simulink model "CHB_3phaseCL_SVPWM_Phaseshift"  (R2015a)
settings: Solver=ode45  StartTime=0.0  StopTime=0.2  MaxStep=0.00001  MinStep=0.000001  RelTol=1e-3
libraries: powerlib x33, powerlib_meascontrol x3, simulink x3
settings Model: Creator=hp  LastModifiedBy=hp
settings SolverCC: ZeroCrossControl=DisableAll

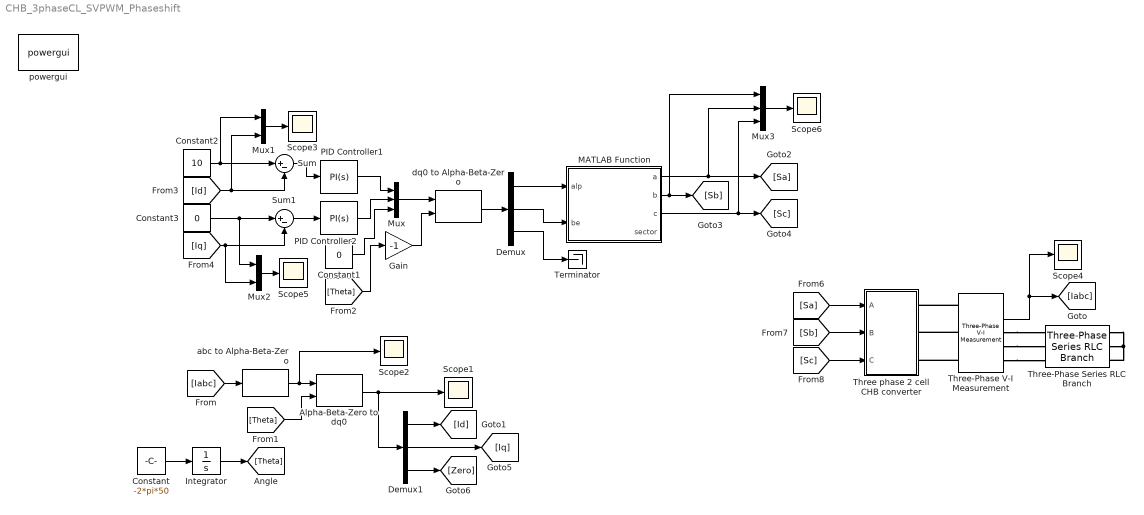
== system CHB_3phaseCL_SVPWM_Phaseshift ==
  Alpha-Beta-Zero to dq0 : powerlib_meascontrol/Transformations/Alpha-Beta-Zero to dq0  Alignment=Aligned with phase A axis
  Constant : Constant  Value=-2*pi*50
  Constant1 : Constant  Value=0
  Constant2 : Constant  Value=10
  Constant3 : Constant  Value=0
  Demux : Demux  Outputs=3
  Demux1 : Demux  Outputs=3
  Gain : Gain  Gain=-1
  Integrator : Integrator
  MATLAB Function : MATLAB Function  TreatAsAtomicUnit=on
  Mux : Mux  Inputs=3
  Mux1 : Mux  Inputs=2
  Mux2 : Mux  Inputs=2
  Mux3 : Mux  Inputs=3
  PID Controller1 : simulink/Continuous/PID Controller  Controller=PI  TimeDomain=Continuous-time  SampleTime=-1  IntegratorMethod=Forward Euler  FilterMethod=Forward Euler  Form=Parallel  UseFilter=on  ControllerParametersSource=internal  P=1  I=3128.4128432425  D=0  N=100  InitialConditionSource=internal  InitialConditionForIntegrator=0  InitialConditionForFilter=0  ExternalReset=none  LimitOutput=off  UpperSaturationLimit=inf  LowerSaturationLimit=-inf  LinearizeAsGain=on  AntiWindupMode=none  Kb=1  TrackingMode=off  Kt=1  PParamMin=[]  PParamMax=[]  IParamMin=[]  IParamMax=[]  DParamMin=[]  DParamMax=[]  NParamMin=[]  NParamMax=[]  KbParamMin=[]  KbParamMax=[]  KtParamMin=[]  KtParamMax=[]  POutMin=[]  POutMax=[]  IOutMin=[]  IOutMax=[]  DOutMin=[]  DOutMax=[]  NOutMin=[]  NOutMax=[]  KbOutMin=[]  KbOutMax=[]  KtOutMin=[]  KtOutMax=[]  IntegratorOutMin=[]  IntegratorOutMax=[]  FilterOutMin=[]  FilterOutMax=[]  SumOutMin=[]  SumOutMax=[]  SumI1OutMin=[]  SumI1OutMax=[]  SumI2OutMin=[]  SumI2OutMax=[]  SumI3OutMin=[]  SumI3OutMax=[]  SumDOutMin=[]  SumDOutMax=[]  SaturationOutMin=[]  SaturationOutMax=[]  IntegratorContinuousStateAttributes=''  IntegratorStateMustResolveToSignalObject=off  IntegratorRTWStateStorageClass=Auto  FilterContinuousStateAttributes=''  FilterStateMustResolveToSignalObject=off  FilterRTWStateStorageClass=Auto  DifferentiatorICPrevScaledInput=0  DifferentiatorOutMin=[]  DifferentiatorOutMax=[]
  PID Controller2 : simulink/Continuous/PID Controller  Controller=PI  TimeDomain=Continuous-time  SampleTime=-1  IntegratorMethod=Forward Euler  FilterMethod=Forward Euler  Form=Parallel  UseFilter=on  ControllerParametersSource=internal  P=1  I=3128.4128432425  D=0  N=100  InitialConditionSource=internal  InitialConditionForIntegrator=0  InitialConditionForFilter=0  ExternalReset=none  LimitOutput=off  UpperSaturationLimit=inf  LowerSaturationLimit=-inf  LinearizeAsGain=on  AntiWindupMode=none  Kb=1  TrackingMode=off  Kt=1  PParamMin=[]  PParamMax=[]  IParamMin=[]  IParamMax=[]  DParamMin=[]  DParamMax=[]  NParamMin=[]  NParamMax=[]  KbParamMin=[]  KbParamMax=[]  KtParamMin=[]  KtParamMax=[]  POutMin=[]  POutMax=[]  IOutMin=[]  IOutMax=[]  DOutMin=[]  DOutMax=[]  NOutMin=[]  NOutMax=[]  KbOutMin=[]  KbOutMax=[]  KtOutMin=[]  KtOutMax=[]  IntegratorOutMin=[]  IntegratorOutMax=[]  FilterOutMin=[]  FilterOutMax=[]  SumOutMin=[]  SumOutMax=[]  SumI1OutMin=[]  SumI1OutMax=[]  SumI2OutMin=[]  SumI2OutMax=[]  SumI3OutMin=[]  SumI3OutMax=[]  SumDOutMin=[]  SumDOutMax=[]  SaturationOutMin=[]  SaturationOutMax=[]  IntegratorContinuousStateAttributes=''  IntegratorStateMustResolveToSignalObject=off  IntegratorRTWStateStorageClass=Auto  FilterContinuousStateAttributes=''  FilterStateMustResolveToSignalObject=off  FilterRTWStateStorageClass=Auto  DifferentiatorICPrevScaledInput=0  DifferentiatorOutMin=[]  DifferentiatorOutMax=[]
  Scope{1..6} (6 alike) : Scope
      Scope1 settings: YMin=-22.5  YMax=7.5
      Scope2 settings: YMin=-25  YMax=25  SaveName=ScopeData2
      Scope3 settings: YMin=-20  YMax=27.5  SaveName=ScopeData3
      Scope4 settings: YMin=-27.5  YMax=27.5  SaveName=ScopeData5
      Scope5 settings: YMin=-25  YMax=0  SaveName=ScopeData4
      Scope6 settings: YMin=-1750  YMax=1750  SaveName=ScopeData6
  Sum : Sum  Inputs=|+-
  Sum1 : Sum  Inputs=|+-
  Terminator : Terminator
  Three phase 2 cell CHB converter : Subsystem  RequirementInfo="{}  %GIDa_28e9eb3f_ab9c_4722_bfe7_30b5ff19310e"
  Three-Phase Series RLC Branch : powerlib/Elements/Three-Phase Series RLC Branch  LConnTagsString=A|B|C  RConnTagsString=A|B|C  BranchType=RLC  Resistance=10  Inductance=10e-3  Capacitance=0  Measurements=None
  Three-Phase V-I Measurement : powerlib/Measurements/Three-Phase V-I Measurement  VoltageMeasurement=phase-to-phase  SetLabelV=off  LabelV=Vabc  Vpu=off  VpuLL=off  CurrentMeasurement=yes  SetLabelI=off  LabelI=Iabc  Ipu=off  Pbase=100e6  Vbase=500e3  OutputType=Complex  PhasorSimulation=off  PSBequivalent=0
  abc to Alpha-Beta-Zero : powerlib_meascontrol/Transformations/abc to Alpha-Beta-Zero
  dq0 to Alpha-Beta-Zero : powerlib_meascontrol/Transformations/dq0 to Alpha-Beta-Zero  Alignment=Aligned with phase A axis
  powergui : powerlib/powergui  Priority=1  SimulationMode=Continuous  SolverType=Tustin/Backward Euler (TBE)  SampleTime=2e-6  frequency=60  SPID=off  DisableSnubberDevices=off  DisableRonSwitches=off  DisableVfSwitches=off  SwTol=0  DisplayEquations=off  Interpol=off  methode=off  Ts=100  FunctionMessages=off  echomessages=off  HookPort=off  EnableUseOfTLC=off  x0status=blocks  frequencyindice=0  Pbase=100e6  ErrMax=1e-4  Iterations=50  UnitsV=kV  UnitsW=MW  buscounter=0  RestoreLinks=warning  ResistiveCurrentMeasurement=off  Frange=[0:2:500]  Ylog=off  Xlog=on  ShowGrid=off  save=off  variable=ZData  structure=0  ZoomFFT=off  StartTime=0.0  cycles=1  DisplayStyle=1  fundamental=60  FreqAxis=off  MaxFrequency=1000  frequencyindicesteady=1  RmsSteady=1  display=off
  wires:
  MATLAB Function/1(a) -> Mux3/2, [Sa]
  MATLAB Function/2(b) -> Mux3/1, [Sb]
  MATLAB Function/3(c) -> Mux3/3, [Sc]
  Three-Phase V-I Measurement/2 -> Scope4/1, [Iabc]
  [Sa] -> Three phase 2 cell CHB converter/1(A)
  [Sb] -> Three phase 2 cell CHB converter/2(B)
  [Sc] -> Three phase 2 cell CHB converter/3(C)
  [Iabc] -> abc to Alpha-Beta-Zero/1
  Alpha-Beta-Zero to dq0/1 -> Demux1/1, Scope1/1
  Constant/1 -> Integrator/1
  abc to Alpha-Beta-Zero/1 -> Scope2/1, Alpha-Beta-Zero to dq0/1
  Integrator/1 -> [Theta]
  [Theta] -> Alpha-Beta-Zero to dq0/2
  Demux1/1 -> [Id]
  Demux1/2 -> [Iq]
  Demux1/3 -> [Zero]
  Demux/2 -> MATLAB Function/2(be)
  Demux/1 -> MATLAB Function/1(alp)
  dq0 to Alpha-Beta-Zero/1 -> Demux/1
  Mux/1 -> dq0 to Alpha-Beta-Zero/1
  PID Controller1/1 -> Mux/1
  PID Controller2/1 -> Mux/2
  Constant1/1 -> Mux/3
  Sum1/1 -> PID Controller2/1
  Sum/1 -> PID Controller1/1
  Constant3/1 -> Sum1/1, Mux2/1
  [Iq] -> Sum1/2, Mux2/2
  [Id] -> Mux1/2, Sum/2
  Constant2/1 -> Mux1/1, Sum/1
  Mux1/1 -> Scope3/1
  Demux/3 -> Terminator/1
  Mux2/1 -> Scope5/1
  Gain/1 -> dq0 to Alpha-Beta-Zero/2
  [Theta] -> Gain/1
  Mux3/1 -> Scope6/1
  connections:
  Three-Phase Series RLC Branch/RConn1 -- Three-Phase Series RLC Branch/RConn2 -- Three-Phase Series RLC Branch/RConn3
  Three-Phase V-I Measurement/RConn1 -- Three-Phase Series RLC Branch/LConn1
  Three-Phase V-I Measurement/RConn2 -- Three-Phase Series RLC Branch/LConn2
  Three-Phase V-I Measurement/RConn3 -- Three-Phase Series RLC Branch/LConn3
  Three-Phase V-I Measurement/LConn1 -- Three phase 2 cell CHB converter/RConn1
  Three-Phase V-I Measurement/LConn2 -- Three phase 2 cell CHB converter/RConn2
  Three-Phase V-I Measurement/LConn3 -- Three phase 2 cell CHB converter/RConn3

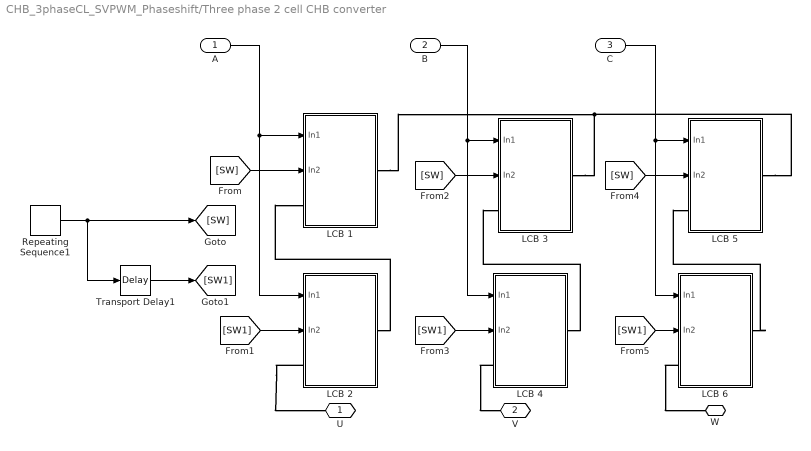
== system CHB_3phaseCL_SVPWM_Phaseshift/Three phase 2 cell CHB converter ==
  A : Inport
  B : Inport  Port=2
  C : Inport  Port=3
  LCB 1 : Subsystem
  LCB 2 : Subsystem
  LCB 3 : Subsystem
  LCB 4 : Subsystem
  LCB 5 : Subsystem
  LCB 6 : Subsystem
  Repeating Sequence1 : simulink/Sources/Repeating Sequence  rep_seq_t=[0 0.5 1]/1000  rep_seq_y=[0 1 0]
  Transport Delay1 : TransportDelay  DelayTime=1/4000
  U : PMIOPort  Port=1  Side=Right
  V : PMIOPort  Port=2  Side=Right
  W : PMIOPort  Port=3  Side=Right
  wires:
  [SW1] -> LCB 2/2(In2)
  [SW1] -> LCB 6/2(In2)
  A/1 -> LCB 2/1(In1), LCB 1/1(In1)
  [SW] -> LCB 3/2(In2)
  Repeating Sequence1/1 -> Transport Delay1/1, [SW]
  C/1 -> LCB 6/1(In1), LCB 5/1(In1)
  [SW] -> LCB 1/2(In2)
  [SW1] -> LCB 4/2(In2)
  Transport Delay1/1 -> [SW1]
  B/1 -> LCB 4/1(In1), LCB 3/1(In1)
  [SW] -> LCB 5/2(In2)
  connections:
  LCB 1/RConn1 -- LCB 5/RConn1 -- LCB 3/RConn1
  LCB 2/RConn1 -- LCB 1/LConn1
  LCB 4/RConn1 -- LCB 3/LConn1
  LCB 2/LConn1 -- U/RConn1
  LCB 6/RConn1 -- LCB 5/LConn1
  LCB 4/LConn1 -- V/RConn1
  LCB 6/LConn1 -- W/RConn1

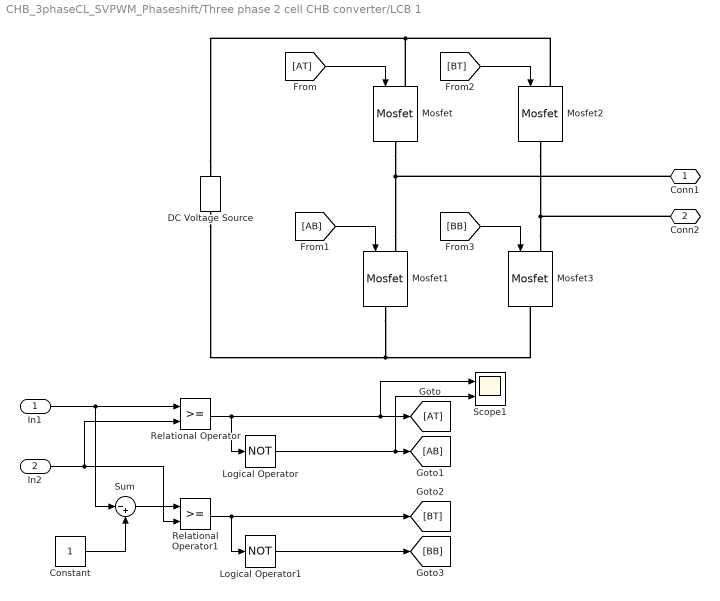
== system CHB_3phaseCL_SVPWM_Phaseshift/Three phase 2 cell CHB converter/LCB 1 ==
  In1 : Inport
  In2 : Inport  Port=2
  Constant : Constant
  DC Voltage Source : powerlib/Electrical Sources/DC Voltage Source  Amplitude=100  Measurements=None
  Logical Operator : Logic  Operator=NOT  Inputs=1  AllPortsSameDT=off  OutDataTypeStr=boolean
  Logical Operator1 : Logic  Operator=NOT  Inputs=1  AllPortsSameDT=off  OutDataTypeStr=boolean
  Mosfet{,1..3} (4 alike) : powerlib/Power Electronics/Mosfet  Ron=0.1  Lon=0  Rd=0.01  Vfd=0  IC=0  Rs=1e5  Cs=inf  Measurements=off
  Relational Operator : RelationalOperator  OutDataTypeStr=boolean
  Relational Operator1 : RelationalOperator  OutDataTypeStr=boolean
  Scope1 : Scope  NumInputPorts=2
      settings: YMin=-80~-5  YMax=80~5
  Sum : Sum  Inputs=|-+
  Conn1 : PMIOPort  Port=1  Side=Right
  Conn2 : PMIOPort  Port=2  Side=Left
  wires:
  Constant/1 -> Sum/2
  In1/1 -> Relational Operator/1, Sum/1
  In2/1 -> Relational Operator/2, Relational Operator1/2
  [BT] -> Mosfet2/1
  [AT] -> Mosfet/1
  [AB] -> Mosfet1/1
  [BB] -> Mosfet3/1
  Logical Operator1/1 -> [BB]
  Relational Operator1/1 -> Logical Operator1/1, [BT]
  Logical Operator/1 -> [AB], Scope1/2
  Relational Operator/1 -> Logical Operator/1, [AT], Scope1/1
  Sum/1 -> Relational Operator1/1
  connections:
  Mosfet1/LConn1 -- Conn1/RConn1 -- Mosfet/RConn1
  DC Voltage Source/RConn1 -- Mosfet/LConn1 -- Mosfet2/LConn1
  Mosfet3/RConn1 -- Mosfet1/RConn1 -- DC Voltage Source/LConn1
  Mosfet3/LConn1 -- Conn2/RConn1 -- Mosfet2/RConn1

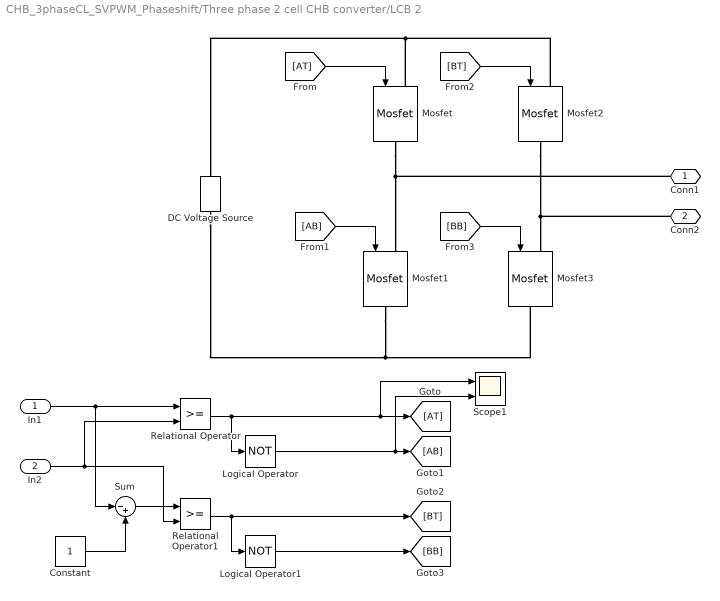
== system CHB_3phaseCL_SVPWM_Phaseshift/Three phase 2 cell CHB converter/LCB 2 ==
  In1 : Inport
  In2 : Inport  Port=2
  Constant : Constant
  DC Voltage Source : powerlib/Electrical Sources/DC Voltage Source  Amplitude=100  Measurements=None
  Logical Operator : Logic  Operator=NOT  Inputs=1  AllPortsSameDT=off  OutDataTypeStr=boolean
  Logical Operator1 : Logic  Operator=NOT  Inputs=1  AllPortsSameDT=off  OutDataTypeStr=boolean
  Mosfet{,1..3} (4 alike) : powerlib/Power Electronics/Mosfet  Ron=0.1  Lon=0  Rd=0.01  Vfd=0  IC=0  Rs=1e5  Cs=inf  Measurements=off
  Relational Operator : RelationalOperator  OutDataTypeStr=boolean
  Relational Operator1 : RelationalOperator  OutDataTypeStr=boolean
  Scope1 : Scope  NumInputPorts=2
      settings: YMin=-80~-5  YMax=80~5
  Sum : Sum  Inputs=|-+
  Conn1 : PMIOPort  Port=1  Side=Right
  Conn2 : PMIOPort  Port=2  Side=Left
  wires:
  Sum/1 -> Relational Operator1/1
  Relational Operator/1 -> Scope1/1, [AT], Logical Operator/1
  Logical Operator/1 -> Scope1/2, [AB]
  Relational Operator1/1 -> [BT], Logical Operator1/1
  Logical Operator1/1 -> [BB]
  [BB] -> Mosfet3/1
  [AB] -> Mosfet1/1
  [AT] -> Mosfet/1
  [BT] -> Mosfet2/1
  In2/1 -> Relational Operator1/2, Relational Operator/2
  In1/1 -> Sum/1, Relational Operator/1
  Constant/1 -> Sum/2
  connections:
  Mosfet2/RConn1 -- Conn2/RConn1 -- Mosfet3/LConn1
  DC Voltage Source/LConn1 -- Mosfet1/RConn1 -- Mosfet3/RConn1
  Mosfet2/LConn1 -- Mosfet/LConn1 -- DC Voltage Source/RConn1
  Mosfet/RConn1 -- Conn1/RConn1 -- Mosfet1/LConn1

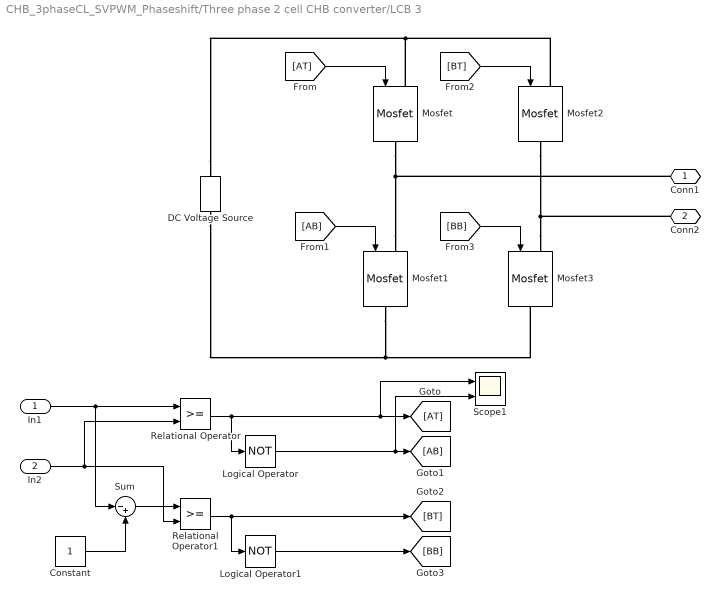
== system CHB_3phaseCL_SVPWM_Phaseshift/Three phase 2 cell CHB converter/LCB 3 ==
  In1 : Inport
  In2 : Inport  Port=2
  Constant : Constant
  DC Voltage Source : powerlib/Electrical Sources/DC Voltage Source  Amplitude=100  Measurements=None
  Logical Operator : Logic  Operator=NOT  Inputs=1  AllPortsSameDT=off  OutDataTypeStr=boolean
  Logical Operator1 : Logic  Operator=NOT  Inputs=1  AllPortsSameDT=off  OutDataTypeStr=boolean
  Mosfet{,1..3} (4 alike) : powerlib/Power Electronics/Mosfet  Ron=0.1  Lon=0  Rd=0.01  Vfd=0  IC=0  Rs=1e5  Cs=inf  Measurements=off
  Relational Operator : RelationalOperator  OutDataTypeStr=boolean
  Relational Operator1 : RelationalOperator  OutDataTypeStr=boolean
  Scope1 : Scope  NumInputPorts=2
      settings: YMin=-80~-5  YMax=80~5
  Sum : Sum  Inputs=|-+
  Conn1 : PMIOPort  Port=1  Side=Right
  Conn2 : PMIOPort  Port=2  Side=Left
  wires:
  Constant/1 -> Sum/2
  In1/1 -> Relational Operator/1, Sum/1
  In2/1 -> Relational Operator/2, Relational Operator1/2
  [BT] -> Mosfet2/1
  [AT] -> Mosfet/1
  [AB] -> Mosfet1/1
  [BB] -> Mosfet3/1
  Logical Operator1/1 -> [BB]
  Relational Operator1/1 -> Logical Operator1/1, [BT]
  Logical Operator/1 -> [AB], Scope1/2
  Relational Operator/1 -> Logical Operator/1, [AT], Scope1/1
  Sum/1 -> Relational Operator1/1
  connections:
  Mosfet1/LConn1 -- Conn1/RConn1 -- Mosfet/RConn1
  DC Voltage Source/RConn1 -- Mosfet/LConn1 -- Mosfet2/LConn1
  Mosfet3/RConn1 -- Mosfet1/RConn1 -- DC Voltage Source/LConn1
  Mosfet3/LConn1 -- Conn2/RConn1 -- Mosfet2/RConn1

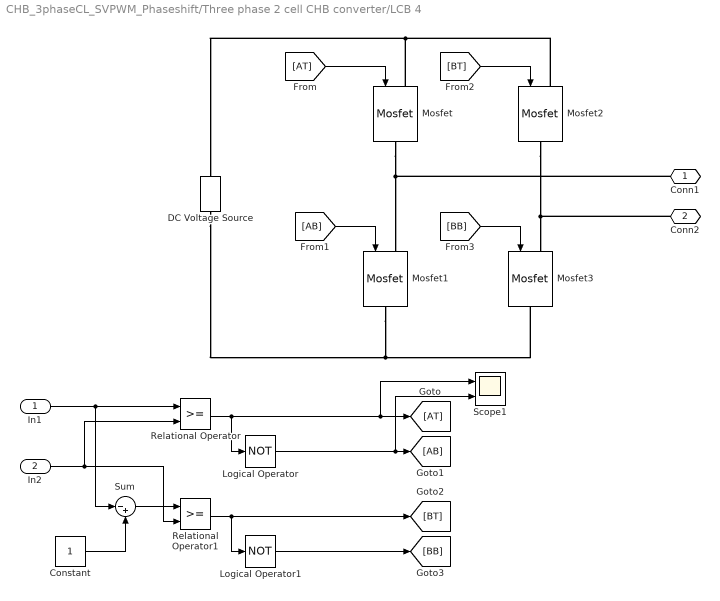
== system CHB_3phaseCL_SVPWM_Phaseshift/Three phase 2 cell CHB converter/LCB 4 ==
  In1 : Inport
  In2 : Inport  Port=2
  Constant : Constant
  DC Voltage Source : powerlib/Electrical Sources/DC Voltage Source  Amplitude=100  Measurements=None
  Logical Operator : Logic  Operator=NOT  Inputs=1  AllPortsSameDT=off  OutDataTypeStr=boolean
  Logical Operator1 : Logic  Operator=NOT  Inputs=1  AllPortsSameDT=off  OutDataTypeStr=boolean
  Mosfet{,1..3} (4 alike) : powerlib/Power Electronics/Mosfet  Ron=0.1  Lon=0  Rd=0.01  Vfd=0  IC=0  Rs=1e5  Cs=inf  Measurements=off
  Relational Operator : RelationalOperator  OutDataTypeStr=boolean
  Relational Operator1 : RelationalOperator  OutDataTypeStr=boolean
  Scope1 : Scope  NumInputPorts=2
      settings: YMin=-80~-5  YMax=80~5
  Sum : Sum  Inputs=|-+
  Conn1 : PMIOPort  Port=1  Side=Right
  Conn2 : PMIOPort  Port=2  Side=Left
  wires:
  Sum/1 -> Relational Operator1/1
  Relational Operator/1 -> Scope1/1, [AT], Logical Operator/1
  Logical Operator/1 -> Scope1/2, [AB]
  Relational Operator1/1 -> [BT], Logical Operator1/1
  Logical Operator1/1 -> [BB]
  [BB] -> Mosfet3/1
  [AB] -> Mosfet1/1
  [AT] -> Mosfet/1
  [BT] -> Mosfet2/1
  In2/1 -> Relational Operator1/2, Relational Operator/2
  In1/1 -> Sum/1, Relational Operator/1
  Constant/1 -> Sum/2
  connections:
  Mosfet2/RConn1 -- Conn2/RConn1 -- Mosfet3/LConn1
  DC Voltage Source/LConn1 -- Mosfet1/RConn1 -- Mosfet3/RConn1
  Mosfet2/LConn1 -- Mosfet/LConn1 -- DC Voltage Source/RConn1
  Mosfet/RConn1 -- Conn1/RConn1 -- Mosfet1/LConn1

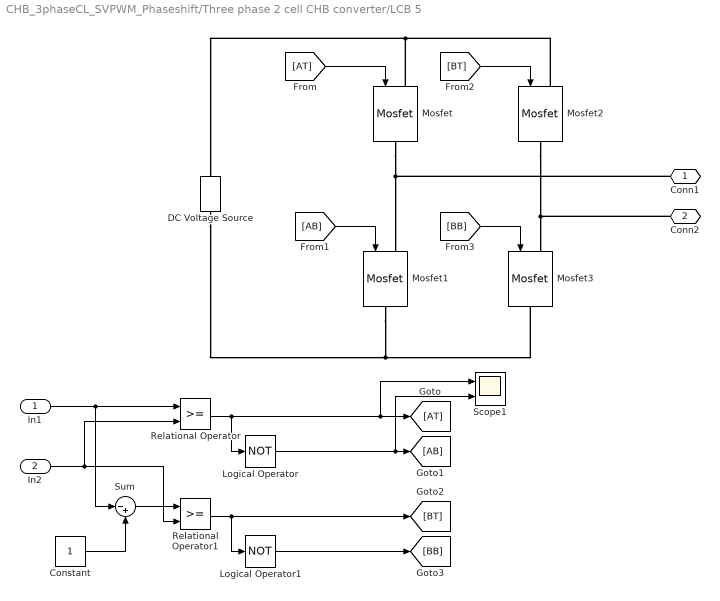
== system CHB_3phaseCL_SVPWM_Phaseshift/Three phase 2 cell CHB converter/LCB 5 ==
  In1 : Inport
  In2 : Inport  Port=2
  Constant : Constant
  DC Voltage Source : powerlib/Electrical Sources/DC Voltage Source  Amplitude=100  Measurements=None
  Logical Operator : Logic  Operator=NOT  Inputs=1  AllPortsSameDT=off  OutDataTypeStr=boolean
  Logical Operator1 : Logic  Operator=NOT  Inputs=1  AllPortsSameDT=off  OutDataTypeStr=boolean
  Mosfet{,1..3} (4 alike) : powerlib/Power Electronics/Mosfet  Ron=0.1  Lon=0  Rd=0.01  Vfd=0  IC=0  Rs=1e5  Cs=inf  Measurements=off
  Relational Operator : RelationalOperator  OutDataTypeStr=boolean
  Relational Operator1 : RelationalOperator  OutDataTypeStr=boolean
  Scope1 : Scope  NumInputPorts=2
      settings: YMin=-80~-5  YMax=80~5
  Sum : Sum  Inputs=|-+
  Conn1 : PMIOPort  Port=1  Side=Right
  Conn2 : PMIOPort  Port=2  Side=Left
  wires:
  Sum/1 -> Relational Operator1/1
  Relational Operator/1 -> Scope1/1, [AT], Logical Operator/1
  Logical Operator/1 -> Scope1/2, [AB]
  Relational Operator1/1 -> [BT], Logical Operator1/1
  Logical Operator1/1 -> [BB]
  [BB] -> Mosfet3/1
  [AB] -> Mosfet1/1
  [AT] -> Mosfet/1
  [BT] -> Mosfet2/1
  In2/1 -> Relational Operator1/2, Relational Operator/2
  In1/1 -> Sum/1, Relational Operator/1
  Constant/1 -> Sum/2
  connections:
  Mosfet2/RConn1 -- Conn2/RConn1 -- Mosfet3/LConn1
  DC Voltage Source/LConn1 -- Mosfet1/RConn1 -- Mosfet3/RConn1
  Mosfet2/LConn1 -- Mosfet/LConn1 -- DC Voltage Source/RConn1
  Mosfet/RConn1 -- Conn1/RConn1 -- Mosfet1/LConn1

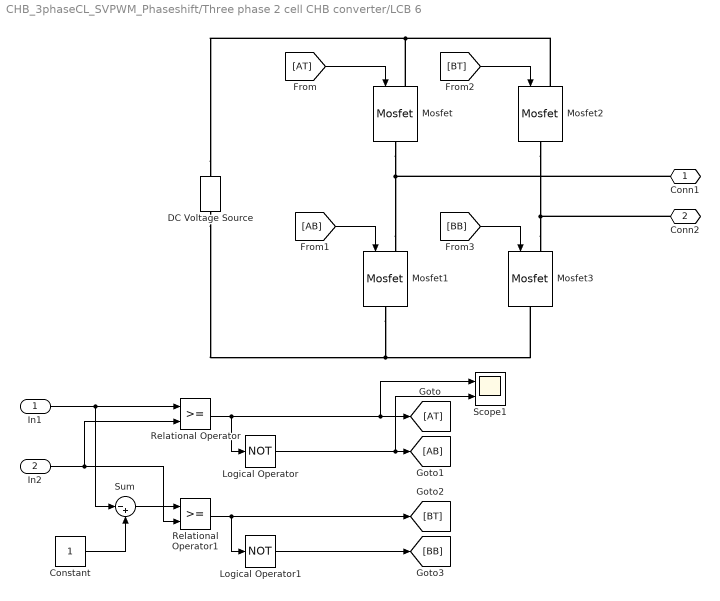
== system CHB_3phaseCL_SVPWM_Phaseshift/Three phase 2 cell CHB converter/LCB 6 ==
  In1 : Inport
  In2 : Inport  Port=2
  Constant : Constant
  DC Voltage Source : powerlib/Electrical Sources/DC Voltage Source  Amplitude=100  Measurements=None
  Logical Operator : Logic  Operator=NOT  Inputs=1  AllPortsSameDT=off  OutDataTypeStr=boolean
  Logical Operator1 : Logic  Operator=NOT  Inputs=1  AllPortsSameDT=off  OutDataTypeStr=boolean
  Mosfet{,1..3} (4 alike) : powerlib/Power Electronics/Mosfet  Ron=0.1  Lon=0  Rd=0.01  Vfd=0  IC=0  Rs=1e5  Cs=inf  Measurements=off
  Relational Operator : RelationalOperator  OutDataTypeStr=boolean
  Relational Operator1 : RelationalOperator  OutDataTypeStr=boolean
  Scope1 : Scope  NumInputPorts=2
      settings: YMin=-80~-5  YMax=80~5
  Sum : Sum  Inputs=|-+
  Conn1 : PMIOPort  Port=1  Side=Right
  Conn2 : PMIOPort  Port=2  Side=Left
  wires:
  Constant/1 -> Sum/2
  In1/1 -> Relational Operator/1, Sum/1
  In2/1 -> Relational Operator/2, Relational Operator1/2
  [BT] -> Mosfet2/1
  [AT] -> Mosfet/1
  [AB] -> Mosfet1/1
  [BB] -> Mosfet3/1
  Logical Operator1/1 -> [BB]
  Relational Operator1/1 -> Logical Operator1/1, [BT]
  Logical Operator/1 -> [AB], Scope1/2
  Relational Operator/1 -> Logical Operator/1, [AT], Scope1/1
  Sum/1 -> Relational Operator1/1
  connections:
  Mosfet1/LConn1 -- Conn1/RConn1 -- Mosfet/RConn1
  DC Voltage Source/RConn1 -- Mosfet/LConn1 -- Mosfet2/LConn1
  Mosfet3/RConn1 -- Mosfet1/RConn1 -- DC Voltage Source/LConn1
  Mosfet3/LConn1 -- Conn2/RConn1 -- Mosfet2/RConn1

== matlab function CHB_3phaseCL_SVPWM_Phaseshift/MATLAB Function ==
  data: alp input; a output; be input; b output; c output; sector output
function [a,b,c,sector] = fcn(alp,be)
%#codegen
	sec_a=0,sec_b=0,sec_c=0;
	t_o = 0,ta = 0,tb = 0,tc = 0,tsec = 0;

    sec_a = be;										%Beta;
	sec_b = ((-be/2)+(alp*0.866));			%(-0.5*Beta+(0.866*alpha));
	sec_c = ((-be/2)-(alp*0.866));			%(-0.5*Beta-(0.866*alpha));
    
    if(sec_a>=0)
       if(sec_b>=0)
       												%	sector 1
    		t_o = (1 - (sec_a+sec_b))/2;							%	t_1 = sec_b, t_2 =sec_a
    		ta = sec_a+sec_b+(t_o);
    		tb  = sec_a+(t_o);
    		tc  = (t_o);
            tsec = 1;
       else
            if(sec_c>=0)												%	sector 3
        		t_o = (1 - (sec_a+sec_c))/2;						%	t_1 = sec_a, t_2 =sec_c
        		ta = (t_o);
        		tb = sec_a+sec_c+(t_o);
        		tc = sec_c+(t_o);
                tsec = 3;
            else												%	sector 2
        		t_o = (1 + (sec_c+sec_b))/2;					%	t_1 = -sec_c, t_2 =-sec_b
        		ta = -sec_c+(t_o);
        		tb = -(sec_c+sec_b)+(t_o);
        		tc = (t_o);
                tsec = 2;
            end
       end
    else
       if(sec_b>=0)
           if(sec_c>=0)                                                  %	sector 5
        		t_o = (1 - (sec_c+sec_b))/2; 				%	t_1 = sec_c, t_2 =sec_b
        		ta = sec_b+(t_o);
        		tb = (t_o);
        		tc = sec_c+sec_b+(t_o);
                tsec = 5;
           else                                                  %	sector 6
        		t_o = (1 + (sec_a+sec_c))/2; 				%	t_1 = -sec_a, t_2 =-sec_c
        		ta = -(sec_a+sec_c)+(t_o);
        		tb = (t_o);
        		tc = -sec_a+(t_o);
                tsec = 6;
           end
       else
            if(sec_c>=0)                                      %	sector 4
        		t_o = (1 + (sec_a+sec_b))/2;			%	t_1 = -sec_b, t_2 =-sec_a
        		ta = (t_o);
        		tb = -sec_b+(t_o);
        		tc = -(sec_a+sec_b)+(t_o);
                tsec = 4;
            end
       end
    end
    % output limiter
    if (ta>1)
        ta = 1;
    end
    if (tb>1)
    tb = 1;
    end
    if (tc>1)
    tc = 1;
    end
    if (ta<0)
    ta = 0;
    end
    if (tb<0)
    tb = 0;
    end
    if (tc<0)
    tc = 0;
    end
a = ta;
b = tb;
c = tc;
sector = tsec;
